simulink model "sim_identificacao_08_04_19"  (R2018a)
settings: Solver=ode4  StartTime=0.0  StopTime=100.0  FixedStep=0.01  RelTol=1e-3
libraries: simulink x1
settings Model: Creator=root  LastModifiedBy=root

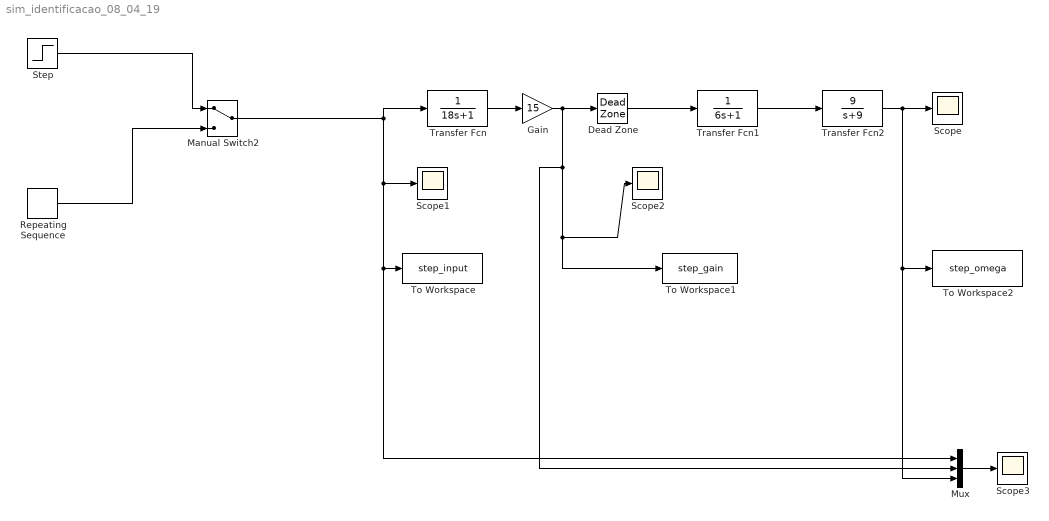
== system sim_identificacao_08_04_19 ==
  Dead Zone : DeadZone  LowerValue=-0.2  UpperValue=0.2  SaturateOnIntegerOverflow=on
  Gain : Gain  Gain=15
  Manual Switch2 : ManualSwitch
  Mux : Mux  Inputs=3
  Repeating Sequence : simulink/Sources/Repeating Sequence  rep_seq_t=[0 2 4 96 98 100]  rep_seq_y=[0 1 0 0 -1 0]
  Scope{,1..3} (4 alike) : Scope
  Step : Step  SampleTime=0
  To Workspace : ToWorkspace  VariableName=step_input  SaveFormat=Timeseries  SampleTime=-1
  To Workspace1 : ToWorkspace  VariableName=step_gain  SaveFormat=Timeseries  SampleTime=-1
  To Workspace2 : ToWorkspace  VariableName=step_omega  SaveFormat=Timeseries  SampleTime=-1
  Transfer Fcn : TransferFcn  Denominator=[18 1]
  Transfer Fcn1 : TransferFcn  Denominator=[6 1]
  Transfer Fcn2 : TransferFcn  Numerator=[9]  Denominator=[1 9]
  wires:
  Manual Switch2/1 -> Transfer Fcn/1, Mux/1, To Workspace/1, Scope1/1
  Transfer Fcn/1 -> Gain/1
  Dead Zone/1 -> Transfer Fcn1/1
  Transfer Fcn1/1 -> Transfer Fcn2/1
  Transfer Fcn2/1 -> Mux/3, To Workspace2/1, Scope/1
  Mux/1 -> Scope3/1
  Gain/1 -> Mux/2, To Workspace1/1, Scope2/1, Dead Zone/1
  Repeating Sequence/1 -> Manual Switch2/2
  Step/1 -> Manual Switch2/1
